simulink library "INT_APP_DD1"  (R2016b)
settings: Solver=VariableStepAuto  StartTime=0.0  StopTime=10.0  RelTol=1e-3
settings Model: Creator=Administrator  LastModifiedBy=Administrator

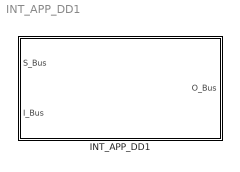
== system INT_APP_DD1 ==
  INT_APP_DD1 : Subsystem

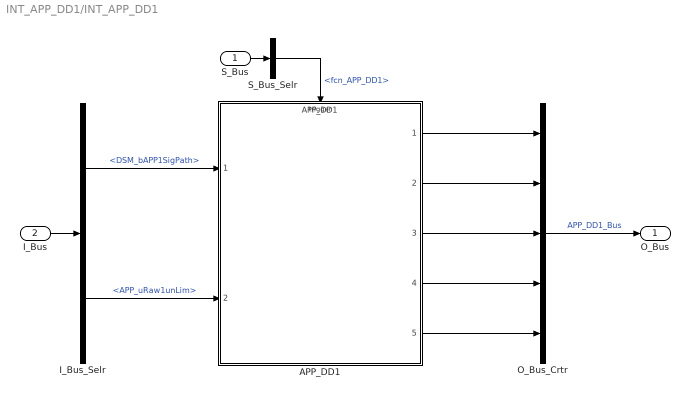
== system INT_APP_DD1/INT_APP_DD1 ==
  S_Bus : Inport
  I_Bus : Inport  Port=2
  APP_DD1 : ModelReference  ModelNameDialog=APP_DD1  SimulationMode=Normal  ModelReferenceVersion=1.20  TriggerPortName=function  TriggerPortTriggerType=function-call  TriggerPortStatesWhenEnabling=held
  I_Bus_Selr : BusSelector  OutputSignals=DSM_bAPP1SigPath,APP_uRaw1unLim
  O_Bus_Crtr : BusCreator  Inputs=5
  S_Bus_Selr : BusSelector  OutputSignals=fcn_APP_DD1
  O_Bus : Outport
  wires:
  S_Bus_Selr/1 -> APP_DD1/Trigger  "<fcn_APP_DD1>"
  S_Bus/1 -> S_Bus_Selr/1
  I_Bus/1 -> I_Bus_Selr/1
  I_Bus_Selr/1 -> APP_DD1/1  "<DSM_bAPP1SigPath>"
  I_Bus_Selr/2 -> APP_DD1/2  "<APP_uRaw1unLim>"
  O_Bus_Crtr/1 -> O_Bus/1  "APP_DD1_Bus"
  APP_DD1/1 -> O_Bus_Crtr/1
  APP_DD1/2 -> O_Bus_Crtr/2
  APP_DD1/3 -> O_Bus_Crtr/3
  APP_DD1/4 -> O_Bus_Crtr/4
  APP_DD1/5 -> O_Bus_Crtr/5
